simulink library "linearizationPlant_cl"  (R2018b)
settings: Solver=VariableStepAuto  StartTime=0.0  StopTime=10.0  RelTol=1e-3
undefined symbols (not defined in the file): DiscIntNeverNeededParam, initialHeading_deg, initialPathPosition_none, initialSpeed_mPs, initialXPosition_m, initialYPosition_m
libraries: calculatePathSpeed x1, pathProjection_ul x1, stateEquations_ul x1
settings Model: Creator=mcobb  LastModifiedBy=mcobb
settings DebuggingCC: LibraryContextMissingDiagnostic=none
settings SFSimCC: SimUseLocalCustomCode=off
settings RTWCC: RTWUseLocalCustomCode=off

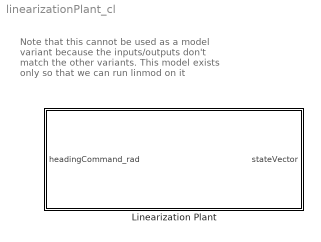
== system linearizationPlant_cl ==
  note: Note that this cannot be used as a
      | model variant because the inputs/outputs
      | don't match the other variants.  This model
      | exists only so that we can run linmod on it
  Linearization Plant : Subsystem  VariantControl=VSS_NONLINEAR_PLNT

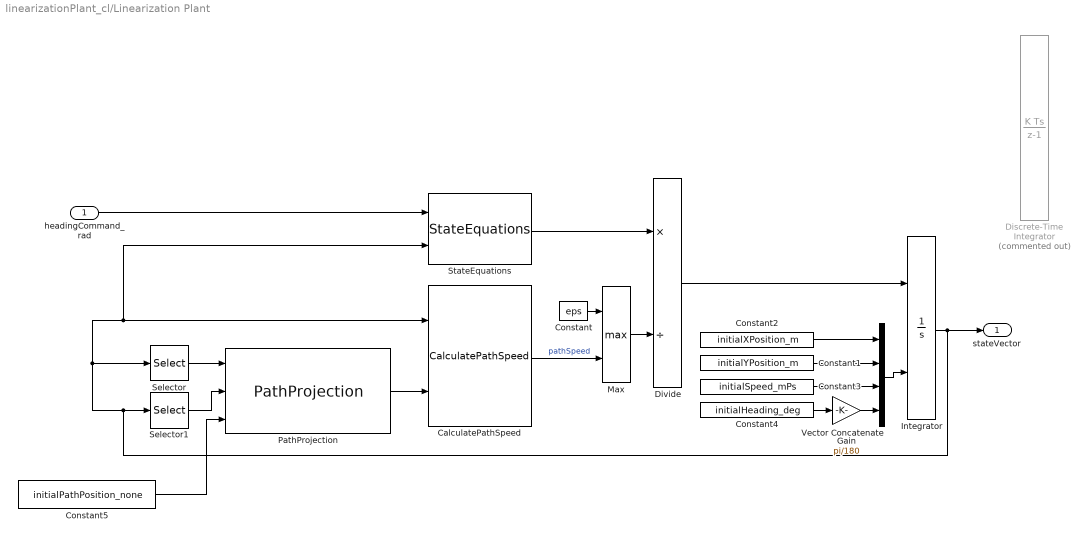
== system linearizationPlant_cl/Linearization Plant ==
  headingCommand_rad : Inport
  CalculatePathSpeed : calculatePathSpeed/CalculatePathSpeed  SystemSampleTime=-1
  Constant : Constant  Value=eps
  Constant1 : Constant  Value=initialYPosition_m
  Constant2 : Constant  Value=initialXPosition_m
  Constant3 : Constant  Value=initialSpeed_mPs
  Constant4 : Constant  Value=initialHeading_deg
  Constant5 : Constant  Value=initialPathPosition_none
  Discrete-Time Integrator : DiscreteIntegrator  Commented=on  InitialConditionSource=external  SampleTime=-1  ICPrevOutput=DiscIntNeverNeededParam  ICPrevScaledInput=DiscIntNeverNeededParam
  Divide : Product  Inputs=*/
  Gain : Gain  Gain=pi/180
  Integrator : Integrator  InitialConditionSource=external
  Max : MinMax  Function=max  Inputs=2
  PathProjection : pathProjection_ul/PathProjection  SystemSampleTime=-1
  Selector : Selector  InputPortWidth=4  IndexOptions=Index vector (dialog)  Indices=1  OutputSizes=1
  Selector1 : Selector  InputPortWidth=4  IndexOptions=Index vector (dialog)  Indices=2  OutputSizes=1
  StateEquations : stateEquations_ul/StateEquations  SystemSampleTime=-1
  Vector Concatenate : Concatenate  NumInputs=4
  stateVector : Outport
  wires:
  headingCommand_rad/1 -> StateEquations/1
  Selector/1 -> PathProjection/1
  Integrator/1 -> Selector1/1, Selector/1, StateEquations/2, CalculatePathSpeed/1, stateVector/1
  Selector1/1 -> PathProjection/2
  PathProjection/1 -> CalculatePathSpeed/2
  StateEquations/1 -> Divide/1
  Max/1 -> Divide/2
  Constant/1 -> Max/1
  CalculatePathSpeed/1 -> Max/2  "pathSpeed"
  Divide/1 -> Integrator/1
  Constant3/1 -> Vector Concatenate/3
  Constant1/1 -> Vector Concatenate/2
  Constant2/1 -> Vector Concatenate/1
  Vector Concatenate/1 -> Integrator/2
  Constant4/1 -> Gain/1
  Gain/1 -> Vector Concatenate/4
  Constant5/1 -> PathProjection/3
